simulink model "tracker2"  (Simulink 6.4)
settings: Solver=ode45  StartTime=0.0  StopTime=10.0  RelTol=1e-3
undefined symbols (not defined in the file): jet
libraries: vipstatistics x2, vipsrcs x2, viptextngfix x1, vipconversions x1, vipsnks x1
settings Model: LastModifiedBy=fnasim

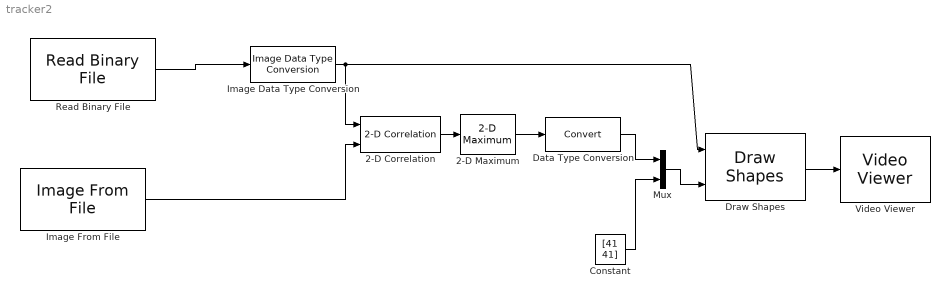
== system tracker2 ==
  2-D Correlation : vipstatistics/2-D Correlation  DialogController=vipDDGCreate  DialogControllerArgs=DataTag0  outSize=Valid  normalize=on  roundingMode=Floor  overflowMode=off
  2-D Maximum : vipstatistics/2-D Maximum  DialogController=dspDDGCreate  DialogControllerArgs=DataTag1  fcn=Index  reset=None  roundingMode=Floor  overflowMode=off
  Constant : Constant  Value=[41 41]  OutDataTypeMode=single  OutDataType=sfix(16)  ConRadixGroup=Use specified scaling  OutScaling=2^0  SampleTime=inf  FramePeriod=inf
  Data Type Conversion : DataTypeConversion  OutDataTypeMode=single
  Draw Shapes : viptextngfix/Draw Shapes  DialogController=vipDDGCreate  DialogControllerArgs=DataTag2  inType=Intensity  shape=Rectangles  fill=off  display=Black  intensity=200  color=[200 255 100]  opacity=0.6  viewport=Entire image  antialiasing=off
  Image Data Type Conversion : vipconversions/Image Data Type Conversion  outDT=single  isSigned=on  wordLen=16  numFracBits=0
  Image From File : vipsrcs/Image From File  DialogController=vipDDGCreate  DialogControllerArgs=DataTag3  SystemSampleTime=-1  FileName=d:\fyp\matlab\misc\cellphone.png  Ts=inf  ImageDataType=single  Signed=on  WordLength=16  sdImageDataType=uint(8)  FractionLengthMode=User-defined  FractionLength=15  OutPortLabels=I
  Mux : Mux  Inputs=2
  Read Binary File : vipsrcs/Read Binary File  DialogController=vipDDGCreate  DialogControllerArgs=DataTag4  FileName=d:\fyp\vid\fas1.bin  loopOrNot=on  numLoops=inf  VideoFormat=Four character codes  FOURCC=GREY  BitStreamFormat=Planar  NumOutputs=3  ComponentOrder=[1 2 3]  Interlaced=off  LineOrdering=Top line first  Ts=1/10  Component1=Y'  Component2=Cb  Component3=Cr  Component4=Alpha  Bits1=8  Bits2=8  Bits3=8  Bits4=8  Rows1=120  Rows2=60  Rows3=60  Rows4=288  Cols1=160  Cols2=80  Cols3=80  Cols4=352  YRows=120  YCols=160  SignedOutput=off  FileEndian=Little endian  OutputEOF=off
  Video Viewer : vipsnks/Video Viewer  inputType=Intensity  useColorMap=off  colormapValue=jet(256);  specRange=off  minInputVal=0  maxInputVal=255  FigPos=[620 632 160 128]  AxisZoom=on  trueSizedOnce=on
  wires:
  2-D Correlation/1 -> 2-D Maximum/1
  2-D Maximum/1 -> Data Type Conversion/1
  Data Type Conversion/1 -> Mux/1
  Constant/1 -> Mux/2
  Mux/1 -> Draw Shapes/2
  Draw Shapes/1 -> Video Viewer/1
  Image Data Type Conversion/1 -> Draw Shapes/1, 2-D Correlation/1
  Image From File/1 -> 2-D Correlation/2
  Read Binary File/1 -> Image Data Type Conversion/1
